simulink model "TARUNPERFORMANCERENEWABLE"  (R2016a)
settings: Solver=VariableStepAuto  StartTime=0.0  StopTime=0.5  RelTol=1e-3
libraries: powerlib x3, simulink x2, re_lib x1
settings Model: Creator=user  LastModifiedBy=user

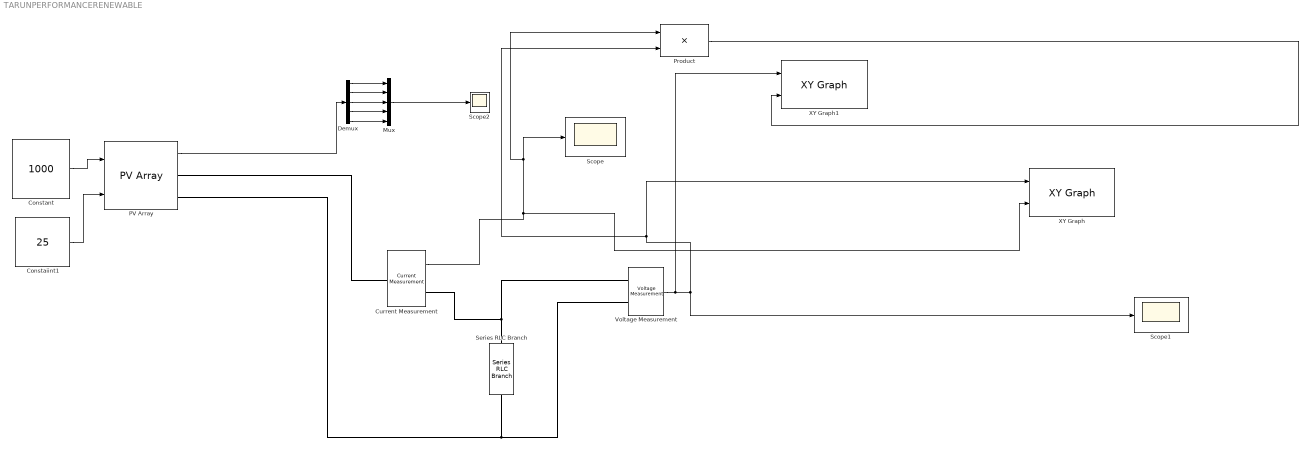
== system TARUNPERFORMANCERENEWABLE ==
  Constaiint1 : Constant  Value=25
  Constant : Constant  Value=1000
  Current Measurement : powerlib/Measurements/Current Measurement  PhasorSimulation=off  OutputType=Complex  PSBequivalent=0
  Demux : Demux  Outputs=5
  Mux : Mux  Inputs=5
  PV Array : re_lib/Solar/PV Array  Npar=10  Nser=10  PlotType=array @ 1000 W/m2 & specified temperatures  S_vec="[ 1000  500  100 ]"  Temp_C_vec="[ 25  ]"  ModuleName=SunPower SER-220P  PlotWhenSelected=off  Pm=219.9716  Ncell=60  Voc=36.3  Isc=8.3  Vm=29.02  Im=7.58  beta_Voc_pc=-0.35501  alpha_Isc_pc=0.043795  beta_Voc=-0.12887  alpha_Isc=0.003635  IL=8.3331  I0=2.2787e-10  nI=0.97003  Rsh=95.1262  Rs=0.37924  BAL=off  Tc=1e-6  Tfilter=5e-5
  Product : Product
  Scope : Scope
  Scope1 : Scope
  Scope2 : Scope
  Series RLC Branch : powerlib/Elements/Series RLC Branch  LConnTagsString=__new0  RConnTagsString=__new0  BranchType=C  Resistance=1  Inductance=1e-3  SetiL0=off  InitialCurrent=0  Capacitance=1000e-6  Setx0=off  InitialVoltage=0  Measurements=None
  Voltage Measurement : powerlib/Measurements/Voltage Measurement  PhasorSimulation=off  OutputType=Complex  PSBequivalent=0
  XY Graph : simulink/Sinks/XY Graph  xmin=0  xmax=4000  ymin=0  ymax=70000  st=-1
  XY Graph1 : simulink/Sinks/XY Graph  xmin=0  xmax=4000  ymin=0  ymax=180000000  st=-1
  wires:
  Constant/1 -> PV Array/1
  Constaiint1/1 -> PV Array/2
  Current Measurement/1 -> Product/1, Scope/1, XY Graph/2
  Voltage Measurement/1 -> XY Graph1/1, Product/2, XY Graph/1, Scope1/1
  PV Array/1 -> Demux/1
  Demux/1 -> Mux/1
  Demux/2 -> Mux/2
  Demux/3 -> Mux/3
  Demux/4 -> Mux/4
  Demux/5 -> Mux/5
  Mux/1 -> Scope2/1
  Product/1 -> XY Graph1/2
  connections:
  PV Array/RConn1 -- Current Measurement/LConn1
  Current Measurement/RConn1 -- Voltage Measurement/LConn1 -- Series RLC Branch/LConn1
  Voltage Measurement/LConn2 -- PV Array/RConn2 -- Series RLC Branch/RConn1
